simulink model "discrete_triggerred_subsystem"  (R2018a)
settings: Solver=VariableStepAuto  StartTime=0.0  StopTime=20  RelTol=1e-3
settings Model: Creator=BEAR  LastModifiedBy=BEAR

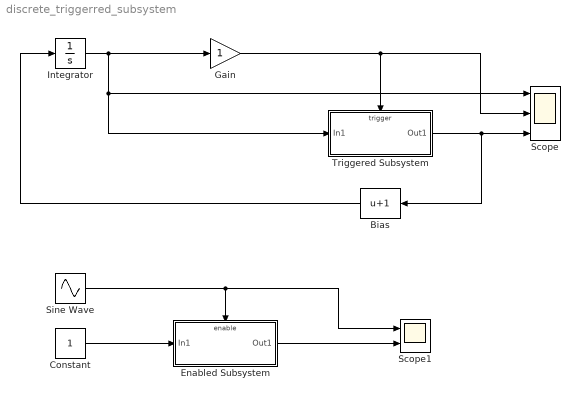
== system discrete_triggerred_subsystem ==
  Bias : Bias  Bias=1
  Constant : Constant
  Enabled Subsystem : Subsystem  TreatAsAtomicUnit=on
  Gain : Gain  SampleTime=1
  Integrator : Integrator  InitialCondition=-1
  Scope : Scope  NumInputPorts=3
  Scope1 : Scope  NumInputPorts=2
  Sine Wave : Sin  SampleTime=0
  Triggered Subsystem : Subsystem  TreatAsAtomicUnit=on
  wires:
  Gain/1 -> Scope/2, Triggered Subsystem/Trigger
  Triggered Subsystem/1(Out1) -> Scope/3, Bias/1
  Bias/1 -> Integrator/1
  Integrator/1 -> Gain/1, Triggered Subsystem/1(In1), Scope/1
  Sine Wave/1 -> Scope1/1, Enabled Subsystem/Enable
  Constant/1 -> Enabled Subsystem/1(In1)
  Enabled Subsystem/1(Out1) -> Scope1/2

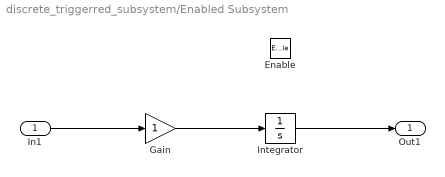
== system discrete_triggerred_subsystem/Enabled Subsystem ==
  In1 : Inport
  Enable : EnablePort
  Gain : Gain  SampleTime=2
  Integrator : Integrator
  Out1 : Outport
  wires:
  Integrator/1 -> Out1/1
  In1/1 -> Gain/1
  Gain/1 -> Integrator/1

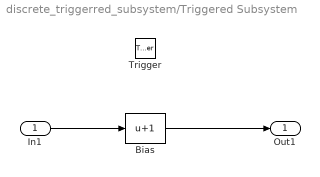
== system discrete_triggerred_subsystem/Triggered Subsystem ==
  In1 : Inport
  Trigger : TriggerPort  VariantControl=Variant
  Bias : Bias  Bias=1
  Out1 : Outport
  wires:
  Bias/1 -> Out1/1
  In1/1 -> Bias/1
